simulink model "pathFollowingWithObstacleAvoidanceExample"  (R2024a)
settings: Solver=VariableStepAuto  StartTime=0.0  StopTime=inf  FixedStep=0.01  RelTol=1e-3  EnableMultiTasking=on
undefined symbols (not defined in the file or in its folder): Angular, Linear
libraries: robotlib x4, robotalgslib x2
settings Model: Creator=The MathWorks, Inc.  LastModifiedBy=WIN
settings SolverCC: AlgebraicLoopSolver=TrustRegion
settings DataIOCC: ReturnWorkspaceOutputs=off
settings DebuggingCC: UnconnectedInputMsg=warning  UnconnectedOutputMsg=warning  UnconnectedLineMsg=warning  ArithmeticOperatorsInVariantConditions=warning
settings ModelReferenceCC: EnableRefExpFcnMdlSchedulingChecks=on
settings SFSimCC: SimUseLocalCustomCode=off  CustomCodeUndefinedFunction=UseInterfaceOnly
settings RTWCC: RTWUseLocalCustomCode=off  GPUComputeCapability=3.5
settings CodeAppCC: StateflowObjectComments=on
settings GRTTargetCC: TargetLangStandard=C89/C90 (ANSI)
settings ConfigComp: CovMetricSettings=dsw  CovSaveCumulativeToWorkspaceVar=on  CovSaveSingleToWorkspaceVar=on  CovExternalEMLEnable=off

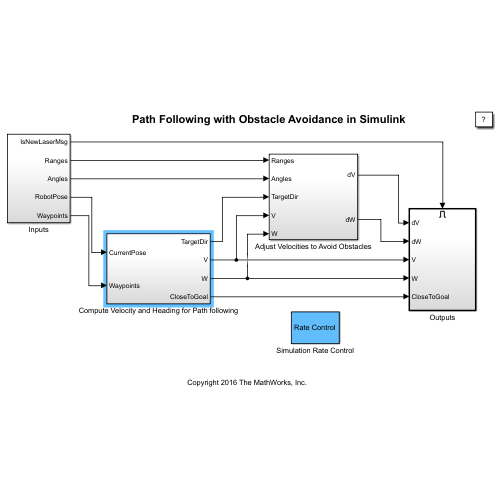
[thumbnail: Simulink's stored preview of the top-level diagram]
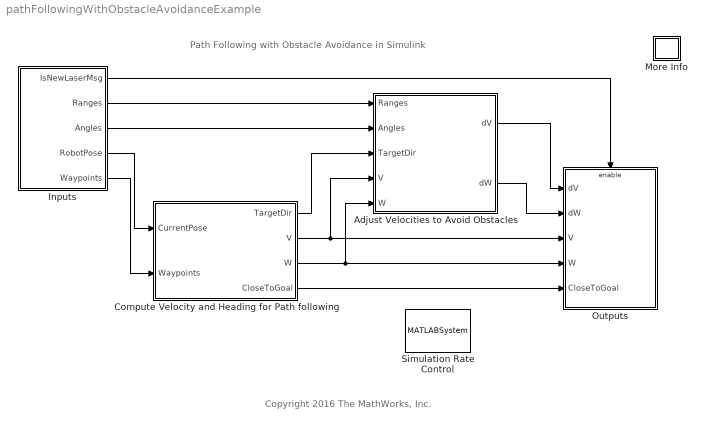
== system pathFollowingWithObstacleAvoidanceExample ==
  note: Path Following with Obstacle Avoidance in Simulink
  note: Copyright 2016 The MathWorks, Inc.
  Adjust Velocities to Avoid Obstacles : Subsystem
  Compute Velocity and Heading for Path following : Subsystem
  Inputs : Subsystem
  More Info : Subsystem
      settings: OpenFcn=showdemo(bdroot(gcb))
      mask Display: disp('?')
  Outputs : Subsystem
  Simulation Rate Control : MATLABSystem  System=ExampleHelperSimulationRateControl  SampleTime=0.02
      mask Type: ExampleHelperSimulationRateControl
      mask Display: disp('Rate Control');
  wires:
  Compute Velocity and Heading for Path following/2(V) -> Outputs/3(V), Adjust Velocities to Avoid Obstacles/4(V)
  Compute Velocity and Heading for Path following/1(TargetDir) -> Adjust Velocities to Avoid Obstacles/3(TargetDir)
  Inputs/2(Ranges) -> Adjust Velocities to Avoid Obstacles/1(Ranges)
  Inputs/3(Angles) -> Adjust Velocities to Avoid Obstacles/2(Angles)
  Inputs/1(IsNewLaserMsg) -> Outputs/Enable
  Inputs/4(RobotPose) -> Compute Velocity and Heading for Path following/1(CurrentPose)
  Inputs/5(Waypoints) -> Compute Velocity and Heading for Path following/2(Waypoints)
  Compute Velocity and Heading for Path following/3(W) -> Outputs/4(W), Adjust Velocities to Avoid Obstacles/5(W)
  Adjust Velocities to Avoid Obstacles/1(dV) -> Outputs/1(dV)
  Adjust Velocities to Avoid Obstacles/2(dW) -> Outputs/2(dW)
  Compute Velocity and Heading for Path following/4(CloseToGoal) -> Outputs/5(CloseToGoal)

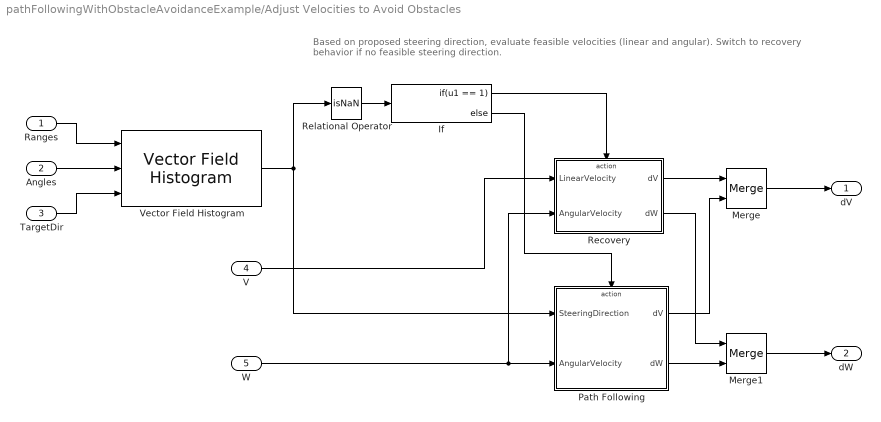
== system pathFollowingWithObstacleAvoidanceExample/Adjust Velocities to Avoid Obstacles ==
  note: Based on proposed steering direction, evaluate feasible velocities (linear and angular).
      | 				Switch to recovery behavior if no feasible steering direction.
  Ranges : Inport
  Angles : Inport  Port=2
  TargetDir : Inport  Port=3
  V : Inport  Port=4
  W : Inport  Port=5
  If : If  IfExpression=u1 == 1
  Merge : Merge
  Merge1 : Merge
  Path Following : Subsystem  TreatAsAtomicUnit=on
  Recovery : Subsystem  TreatAsAtomicUnit=on
  Relational Operator : RelationalOperator  Operator=isNaN  OutDataTypeStr=boolean  RndMeth=Simplest  InputSameDT=off
  Vector Field Histogram : robotalgslib/Vector Field Histogram  NumAngularSectors=180  DistanceLimits=[ 0.05, 3 ]  HistogramThresholds=[ 2, 7 ]  RobotRadius=0.2  SafetyDistance=0.1  MinTurningRadius=0.2  SimulateUsing=Code generation  TargetDirectionWeight=5  CurrentDirectionWeight=2  PreviousDirectionWeight=2
  dV : Outport  VectorParamsAs1DForOutWhenUnconnected=off
  dW : Outport  Port=2  VectorParamsAs1DForOutWhenUnconnected=off
  wires:
  Merge1/1 -> dW/1
  V/1 -> Recovery/1(LinearVelocity)
  Vector Field Histogram/1 -> Relational Operator/1, Path Following/1(SteeringDirection)
  W/1 -> Recovery/2(AngularVelocity), Path Following/2(AngularVelocity)
  Relational Operator/1 -> If/1
  Angles/1 -> Vector Field Histogram/2
  Merge/1 -> dV/1
  TargetDir/1 -> Vector Field Histogram/3
  Ranges/1 -> Vector Field Histogram/1
  If/1 -> Recovery/Action
  If/2 -> Path Following/Action
  Recovery/2(dW) -> Merge1/1
  Path Following/2(dW) -> Merge1/2
  Recovery/1(dV) -> Merge/1
  Path Following/1(dV) -> Merge/2

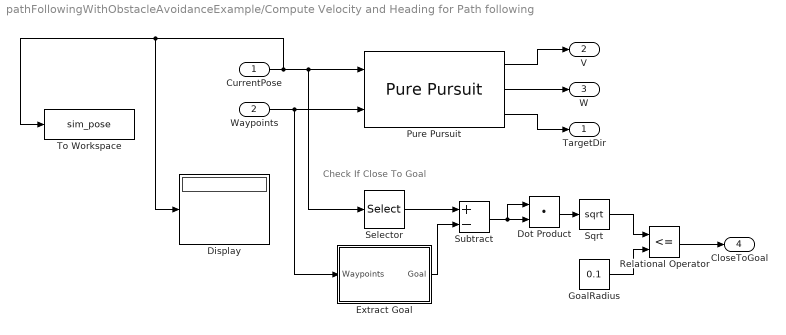
== system pathFollowingWithObstacleAvoidanceExample/Compute Velocity and Heading for Path following ==
  note: Check If Close To Goal
  CurrentPose : Inport
  Waypoints : Inport  Port=2
  " Extract Goal" : MATLAB Function  TreatAsAtomicUnit=on
  Display : Display
  Dot Product : DotProduct  OutDataTypeStr=Inherit: Inherit via internal rule
  GoalRadius : Constant  Value=0.1
  Pure Pursuit : robotalgslib/Pure Pursuit  DesiredLinearVelocityPort=off  DesiredLinearVelocity=0.3  MaxAngularVelocity=1.0  LookaheadDistancePort=off  LookaheadDistance=2.0  TargetDirPort=on  SimulateUsing=Code generation
  Relational Operator : RelationalOperator  Operator=<=  OutDataTypeStr=boolean  RndMeth=Simplest  InputSameDT=off
  Selector : Selector  InputPortWidth=3  IndexOptions=Index vector (dialog)  Indices=[1 2]  OutputSizes=1
  Sqrt : Sqrt
  Subtract : Sum  Inputs=+-
  To Workspace : ToWorkspace  VariableName=sim_pose  SampleTime=-1
      settings: Save2DSignal=2-D array (concatenate along first dimension)
  TargetDir : Outport  VectorParamsAs1DForOutWhenUnconnected=off
  V : Outport  Port=2  VectorParamsAs1DForOutWhenUnconnected=off
  W : Outport  Port=3  VectorParamsAs1DForOutWhenUnconnected=off
  CloseToGoal : Outport  Port=4  VectorParamsAs1DForOutWhenUnconnected=off
  wires:
  Pure Pursuit/3 -> TargetDir/1
  Pure Pursuit/2 -> W/1
  Pure Pursuit/1 -> V/1
  " Extract Goal"/1(Goal) -> Subtract/2
  Waypoints/1 -> " Extract Goal"/1(Waypoints), Pure Pursuit/2
  Relational Operator/1 -> CloseToGoal/1
  GoalRadius/1 -> Relational Operator/2
  Selector/1 -> Subtract/1
  Dot Product/1 -> Sqrt/1
  Sqrt/1 -> Relational Operator/1
  Subtract/1 -> Dot Product/1, Dot Product/2
  CurrentPose/1 -> To Workspace/1, Display/1, Selector/1, Pure Pursuit/1

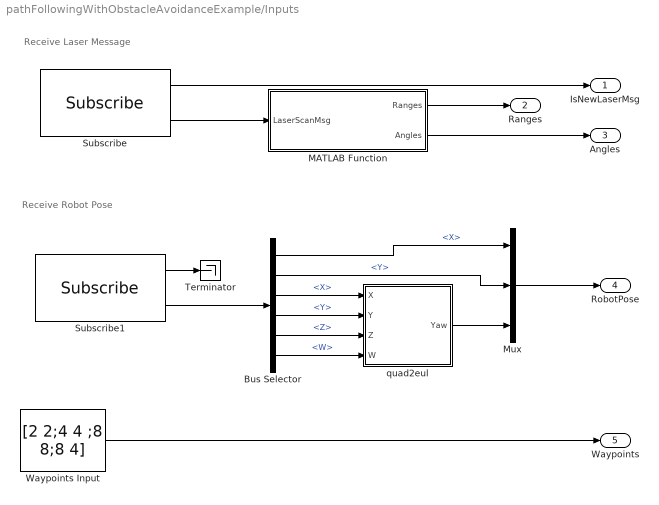
== system pathFollowingWithObstacleAvoidanceExample/Inputs ==
  note: Receive Robot Pose
  note: Receive Laser Message
  Bus Selector : BusSelector  OutputSignals=Pose.Pose.Position.X,Pose.Pose.Position.Y,Pose.Pose.Orientation.X,Pose.Pose.Orientation.Y,Pose.Pose.Orientation.Z,Pose.Pose.Orientation.W
  MATLAB Function : MATLAB Function  TreatAsAtomicUnit=on
  Mux : Mux  Inputs=3
  Subscribe : robotlib/Subscribe  topicSource=Select from ROS network  topic=/scan  messageType=sensor_msgs/LaserScan  SampleTime=-1  legacyBusStruct=off  messageQueueLength=1
  Subscribe1 : robotlib/Subscribe  topicSource=Select from ROS network  topic=/ground_truth_pose  messageType=nav_msgs/Odometry  SampleTime=-1  legacyBusStruct=off  messageQueueLength=1
  Terminator : Terminator
  Waypoints Input : Constant  Value=[2 2;4 4 ;8 8;8 4]  OutDataTypeStr=double  SampleTime=1
  quad2eul : MATLAB Function  TreatAsAtomicUnit=on
  IsNewLaserMsg : Outport  VectorParamsAs1DForOutWhenUnconnected=off
  Ranges : Outport  Port=2  VectorParamsAs1DForOutWhenUnconnected=off
  Angles : Outport  Port=3  VectorParamsAs1DForOutWhenUnconnected=off
  RobotPose : Outport  Port=4  VectorParamsAs1DForOutWhenUnconnected=off
  Waypoints : Outport  Port=5  VectorParamsAs1DForOutWhenUnconnected=off
  wires:
  Waypoints Input/1 -> Waypoints/1
  Subscribe/2 -> MATLAB Function/1(LaserScanMsg)
  quad2eul/1(Yaw) -> Mux/3
  Subscribe1/2 -> Bus Selector/1
  Bus Selector/3 -> quad2eul/1(X)  "<X>"
  Subscribe1/1 -> Terminator/1
  Bus Selector/2 -> Mux/2  "<Y>"
  Bus Selector/5 -> quad2eul/3(Z)  "<Z>"
  Bus Selector/4 -> quad2eul/2(Y)  "<Y>"
  Bus Selector/1 -> Mux/1  "<X>"
  Bus Selector/6 -> quad2eul/4(W)  "<W>"
  MATLAB Function/1(Ranges) -> Ranges/1
  MATLAB Function/2(Angles) -> Angles/1
  Subscribe/1 -> IsNewLaserMsg/1
  Mux/1 -> RobotPose/1

== system pathFollowingWithObstacleAvoidanceExample/More Info ==

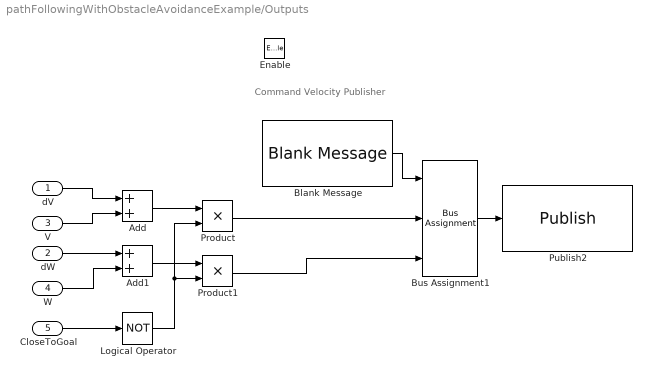
== system pathFollowingWithObstacleAvoidanceExample/Outputs ==
  note: Command Velocity Publisher
  dV : Inport
  dW : Inport  Port=2
  V : Inport  Port=3
  W : Inport  Port=4
  CloseToGoal : Inport  Port=5
  Enable : EnablePort
  Add : Sum
  Add1 : Sum
  Blank Message : robotlib/Blank Message  messageClass=Message  entityType=geometry_msgs/Twist  messageType=geometry_msgs/Twist  SampleTime=inf  legacyBusStruct=off
  Bus Assignment1 : BusAssignment  DialogController=Simulink.DDGSource_BusAssignment  AssignedSignals=Linear.X,Angular.Z
  Logical Operator : Logic  Operator=NOT  AllPortsSameDT=off  OutDataTypeStr=boolean
  Product : Product
  Product1 : Product
  Publish2 : robotlib/Publish  topicSource=Select from ROS network  topic=/mobile_base/commands/velocity  messageType=geometry_msgs/Twist  legacyBusStruct=off  messageQueueLength=105
  wires:
  V/1 -> Add/2
  W/1 -> Add1/2
  dV/1 -> Add/1
  dW/1 -> Add1/1
  CloseToGoal/1 -> Logical Operator/1
  Add/1 -> Product/1
  Add1/1 -> Product1/1
  Product1/1 -> Bus Assignment1/3
  Product/1 -> Bus Assignment1/2
  Blank Message/1 -> Bus Assignment1/1
  Bus Assignment1/1 -> Publish2/1
  Logical Operator/1 -> Product1/2, Product/2

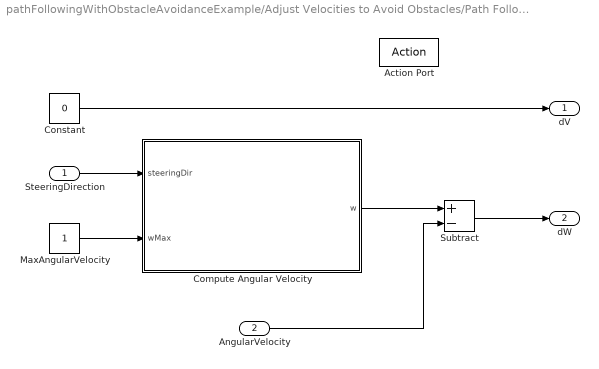
== system pathFollowingWithObstacleAvoidanceExample/Adjust Velocities to Avoid Obstacles/Path Following ==
  SteeringDirection : Inport
  AngularVelocity : Inport  Port=2
  Action Port : ActionPort  ActionPortLabel=else
  Compute Angular Velocity : MATLAB Function  TreatAsAtomicUnit=on
  Constant : Constant  Value=0
  MaxAngularVelocity : Constant
  Subtract : Sum  Inputs=+-
  dV : Outport  VectorParamsAs1DForOutWhenUnconnected=off
  dW : Outport  Port=2  VectorParamsAs1DForOutWhenUnconnected=off
  wires:
  Constant/1 -> dV/1
  MaxAngularVelocity/1 -> Compute Angular Velocity/2(wMax)
  SteeringDirection/1 -> Compute Angular Velocity/1(steeringDir)
  Subtract/1 -> dW/1
  Compute Angular Velocity/1(w) -> Subtract/1
  AngularVelocity/1 -> Subtract/2

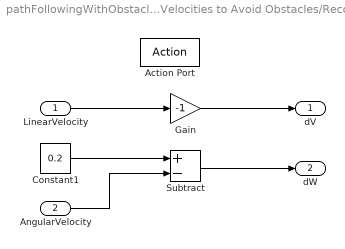
== system pathFollowingWithObstacleAvoidanceExample/Adjust Velocities to Avoid Obstacles/Recovery ==
  LinearVelocity : Inport
  AngularVelocity : Inport  Port=2
  Action Port : ActionPort  ActionPortLabel=if(u1 == 1)
  Constant1 : Constant  Value=0.2
  Gain : Gain  Gain=-1
  Subtract : Sum  Inputs=+-
  dV : Outport  VectorParamsAs1DForOutWhenUnconnected=off
  dW : Outport  Port=2  VectorParamsAs1DForOutWhenUnconnected=off
  wires:
  LinearVelocity/1 -> Gain/1
  Gain/1 -> dV/1
  Constant1/1 -> Subtract/1
  AngularVelocity/1 -> Subtract/2
  Subtract/1 -> dW/1

== matlab function pathFollowingWithObstacleAvoidanceExample/Inputs/quad2eul ==
  data: X input; Yaw output; Y input; Z input; W input
function Yaw = quat2eulBlk(X, Y, Z, W)
%#codegen

eularAngles = quat2eul([W, X, Y, Z]);
Yaw = eularAngles(1);

== matlab function pathFollowingWithObstacleAvoidanceExample/Inputs/MATLAB Function ==
  data: LaserScanMsg input; Ranges output; Angles output
function [Ranges, Angles] = ExtractRangeData(LaserScanMsg)
%#codegen

% Extract Range information
Ranges = double(LaserScanMsg.Ranges);

% Construct Angles vector using AngleMin and AngleIncrement from sensor
% reading.
angMin = double(LaserScanMsg.AngleMin);
angIncrement = double(LaserScanMsg.AngleIncrement);

numReadings = numel(Ranges);
rawAngles = angMin + (0:numReadings-1)' * angIncrement;

% Wrap the angles to the (-pi,pi] interval.
Angles = robotics.internal.wrapToPi(double(rawAngles));

== matlab function pathFollowingWithObstacleAvoidanceExample/Compute Velocity and Heading for Path following/ Extract Goal ==
  data: Waypoints input; Goal output
function Goal = extractGoal(Waypoints)
%#codegen
b = isnan(Waypoints);
[rows,~] = find(b);
ridx = setdiff(1:size(Waypoints,1), sort(rows));
Goal = [Waypoints(ridx(end), 1) Waypoints(ridx(end), 2)];

== matlab function pathFollowingWithObstacleAvoidanceExample/Adjust Velocities to Avoid Obstacles/Path Following/Compute Angular Velocity ==
  data: steeringDir input; w output; wMax input
function w = exampleHelperComputeAngularVelocity(steeringDir, wMax)
%EXAMPLEHELPERCOMPUTEANGULARVELOCITY Compute angular velocity
%   W = exampleHelperComputeAngularVelocity(STEERINGDIR)
%   returns the angular velocity W for a differential drive robot in radians
%   per second for a given steering direction STEERINGDIR in the robot's
%   coordinate frame in radians.
%
%   W = exampleHelperComputeAngularVelocity(STEERINGDIR, WMAX)
%   returns the angular velocity W for a differential drive robot in radians
%   per second for a given steering direction STEERINGDIR in the robot's
%   coordinate frame in radians and maximum angular velocity WMAX in
%   radians per second. The output angular velocity is saturated based on
%   the WMAX.
%
%   Example:
%       
%       w = exampleHelperComputeAngularVelocity(0.2, 1);

% Copyright 2015 The MathWorks, Inc.

%#codegen
%#ok<*EMCA>

% Allow variable input arguments
if nargin == 1   
    wMax = inf;
end

validateattributes(steeringDir, {'double'},{'real'},...
    'exampleHelperComputeAngularVelocity', 'STEERINGDIR', 1);
validateattributes(wMax, {'double'},{'real', 'positive'},...
    'exampleHelperComputeAngularVelocity', 'WMAX', 2);

% Computing in robot's coordinate frame
curPose = [0 0 0];

% The following computation is similar to robotics.PurePursuit
lookaheadPoint = [cos(steeringDir), sin(steeringDir)];
slope = atan2((lookaheadPoint(2) - curPose(2)), ...
    (lookaheadPoint(1) - curPose(1)));
alpha = angdiff(curPose(3), slope);

% Angular velocity command for a differential drive robot is
% equal to the desired curvature to be followed by the robot.

w = (2*sin(alpha));

% Pick a constant rotation when robot is facing in the opposite
% direction of the path
if abs(abs(alpha) - pi) < 1e-12
    w = sign(w)*1;
end

if abs(w) > wMax
    w = sign(w)*wMax;
end

end
